simulink model "dsm_l1_sim"  (Simulink 10.0)
settings: Solver=FixedStepDiscrete  StartTime=0.0  StopTime=10  RelTol=1e-3  AbsTol=1e-6
undefined symbols (not defined in the file): a, b, c, g, Ts
libraries: dspmlti4 x3
settings Model: Creator=mimeiners  LastModifiedBy=Aishwarya
settings SolverCC: AutoScaleAbsTol=off
settings DataIOCC: SaveFormat=Dataset  SignalLoggingSaveFormat=ModelDataLogs  SignalLoggingName=sigsOut
settings OptimizationCC: BooleanDataType=off  LifeSpan=auto
settings DebuggingCC: SaveWithParameterizedLinksMsg=none  SignalResolutionControl=TryResolveAllWithWarning  MultiTaskDSMMsg=warning  MultiTaskCondExecSysMsg=none  SFUnexpectedBacktrackingDiag=error  SFNoUnconditionalDefaultTransitionDiag=error  SFExecutionAtInitializationDiag=warning  UnderSpecifiedDimensionMsg=warning
settings HardwareCC: TargetUnknown=on
settings RTWCC: TemplateMakefile=grt_vc.tmf
settings CodeAppCC: StateflowObjectComments=off
settings ConfigComp: CovExternalEMLEnable=off

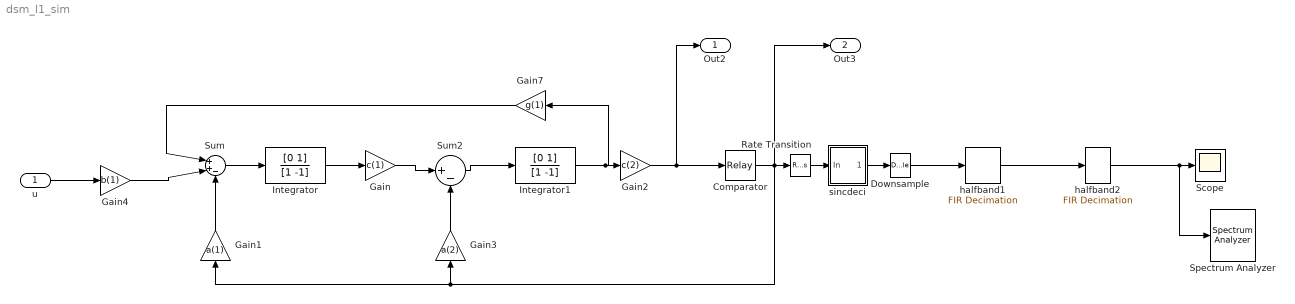
== system dsm_l1_sim ==
  u : Inport
  Comparator : Relay  OffOutputValue=-1
      settings: LockScale=on
  Downsample : DownSample  N=8  RateOptions=Allow multirate processing
  Gain : Gain  Gain=c(1)
  Gain1 : Gain  Gain=a(1)
  Gain2 : Gain  Gain=c(2)
  Gain3 : Gain  Gain=a(2)
  Gain4 : Gain  Gain=b(1)
  Gain7 : Gain  Gain=g(1)
  Integrator : DiscreteFilter  Numerator=[0 1]  Denominator=[1 -1]  SampleTime=Ts
  Integrator1 : DiscreteFilter  Numerator=[0 1]  Denominator=[1 -1]  SampleTime=Ts
  Rate Transition : RateTransition  OutPortSampleTimeOpt=Multiple of input port sample time  OutPortSampleTime=0.1
  Scope : Scope
  Spectrum Analyzer : SpectrumAnalyzer
  Sum : Sum  Inputs=|++-  SaturateOnIntegerOverflow=on  InputSameDT=on  OutDataTypeStr=Inherit: Same as first input
  Sum2 : Sum  Inputs=|+-
  halfband1 : dspmlti4/FIR Decimation  Tag=BlockMethodSubSystem  FilterSource=Dialog parameters  h=[-0.000919098208468256033 -0.00271769602659550002 -0.00248695275983231009 0.00366143838350709017 0.0136509252306624002 0.0173511659010932989 0.00766530619042168036 -0.00655471886964239994 -0.00769678403706536025 0.00610545942139436009 0.0138739157486354008 0.000350861728290910002 -0.0169089254366905015 -0.00890564274915867961 0.0174411295008548989 0.0207450445276099009 -0.0122964942519403 -0.034240865909578401 -0.00103452960557239991 0.0477903055208014974 0.0273630379148479992 -0.0593795188310465988 -0.0823070259292291023 0.0671869094328705063 0.310015177090251004 0.430047880343516986 0.310015177090251004 0.0671869094328705063 -0.0823070259292291023 -0.0593795188310465988 0.0273630379148479992 0.0477903055208014974 -0.00103452960557239991 -0.034240865909578401 -0.0122964942519403 0.0207450445276099009 0.0174411295008548989 -0.00890564274915867961 -0.0169089254366905015 0.000350861728290910002 0.0138739157486354008 0.00610545942139436009 -0.00769678403706536025 -0.00655471886964239994 0.00766530619042168036 0.0173511659010932989 0.0136509252306624002 0.00366143838350709017 -0.00248695275983231009 -0.00271769602659550002 -0.000919098208468256033]  D=4  filtStruct=Direct form  FilterObject=FDECIM  framing=Enforce single-rate processing  inputOffset=0  outputBufInitCond=0  roundingMode=Floor  overflowMode=off  firstCoeffDataTypeStr=Inherit: Same word length as input  firstCoeffMin=[]  firstCoeffMax=[]  firstCoeffLastDataTypeStr=Inherit: Same word length as input  outputMin=[]  outputMax=[]
  halfband2 : dspmlti4/FIR Decimation  Tag=BlockMethodSubSystem  FilterSource=Dialog parameters  h=[-0.000919098208468256033 -0.00271769602659550002 -0.00248695275983231009 0.00366143838350709017 0.0136509252306624002 0.0173511659010932989 0.00766530619042168036 -0.00655471886964239994 -0.00769678403706536025 0.00610545942139436009 0.0138739157486354008 0.000350861728290910002 -0.0169089254366905015 -0.00890564274915867961 0.0174411295008548989 0.0207450445276099009 -0.0122964942519403 -0.034240865909578401 -0.00103452960557239991 0.0477903055208014974 0.0273630379148479992 -0.0593795188310465988 -0.0823070259292291023 0.0671869094328705063 0.310015177090251004 0.430047880343516986 0.310015177090251004 0.0671869094328705063 -0.0823070259292291023 -0.0593795188310465988 0.0273630379148479992 0.0477903055208014974 -0.00103452960557239991 -0.034240865909578401 -0.0122964942519403 0.0207450445276099009 0.0174411295008548989 -0.00890564274915867961 -0.0169089254366905015 0.000350861728290910002 0.0138739157486354008 0.00610545942139436009 -0.00769678403706536025 -0.00655471886964239994 0.00766530619042168036 0.0173511659010932989 0.0136509252306624002 0.00366143838350709017 -0.00248695275983231009 -0.00271769602659550002 -0.000919098208468256033]  D=2  filtStruct=Direct form  FilterObject=FDECIM  framing=Enforce single-rate processing  inputOffset=0  outputBufInitCond=0  roundingMode=Floor  overflowMode=off  firstCoeffDataTypeStr=Inherit: Same word length as input  firstCoeffMin=[]  firstCoeffMax=[]  firstCoeffLastDataTypeStr=Inherit: Same word length as input  outputMin=[]  outputMax=[]
  sincdeci : Subsystem  Tag=BlockMethodSubSystem
  Out2 : Outport
  Out3 : Outport  Port=2
  wires:
  Integrator/1 -> Gain/1
  Gain4/1 -> Sum/2
  Gain1/1 -> Sum/3
  Gain2/1 -> Comparator/1, Out2/1
  u/1 -> Gain4/1
  Integrator1/1 -> Gain7/1, Gain2/1
  Gain7/1 -> Sum/1
  Gain/1 -> Sum2/1
  Sum/1 -> Integrator/1
  Gain3/1 -> Sum2/2
  Sum2/1 -> Integrator1/1
  Rate Transition/1 -> sincdeci/1(In)
  sincdeci/1(Out) -> Downsample/1
  Downsample/1 -> halfband1/1
  halfband1/1 -> halfband2/1
  halfband2/1 -> Spectrum Analyzer/1, Scope/1
  Comparator/1 -> Out3/1, Rate Transition/1, Gain3/1, Gain1/1

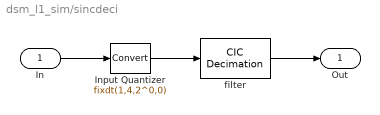
== system dsm_l1_sim/sincdeci ==
  In : Inport
  Input Quantizer : DataTypeConversion  OutDataTypeStr=fixdt(1,4,2^0,0)  SaturateOnIntegerOverflow=on
  filter : dspmlti4/CIC Decimation  filtFrom=Dialog parameters  filtobj=CICDECIM  ftype=Decimator  R=8  M=2  N=2  filterInternals=Specify word lengths  BPS=[22 22 22 22]  FLPS=[15 15 15 15]  outputWordLength=16  outputFracLength=15  launchFVT=off  framing=Maintain input frame rate  RateOptions=Allow multirate processing
      settings: SourceProductName=DSP System Toolbox  SourceProductBaseCode=DS
  Out : Outport
  wires:
  In/1 -> Input Quantizer/1
  Input Quantizer/1 -> filter/1
  filter/1 -> Out/1
